simulink model "simulateur_pendule1"  (R2019b)
settings: Solver=VariableStepAuto  StartTime=0.0  StopTime=30.0  RelTol=1e-3
settings Model: Creator=Morin  LastModifiedBy=Morin

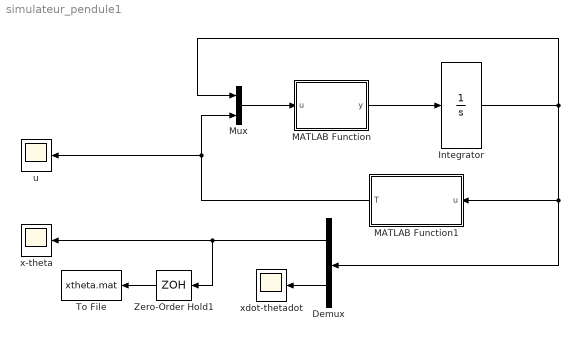
== system simulateur_pendule1 ==
  Demux : Demux  Outputs=2
  Integrator : Integrator  InitialCondition=[0;0.3;0;0]
  MATLAB Function : MATLAB Function  TreatAsAtomicUnit=on
  MATLAB Function1 : MATLAB Function  TreatAsAtomicUnit=on
  Mux : Mux  Inputs=2
  To File : ToFile  Filename=xtheta.mat  SaveFormat=Timeseries  SampleTime=0.01
  Zero-Order Hold1 : ZeroOrderHold  SampleTime=0.01
  u : Scope
  x-theta : Scope
  xdot-thetadot : Scope
  wires:
  MATLAB Function/1(y) -> Integrator/1
  Integrator/1 -> Mux/1, Demux/1, MATLAB Function1/1(u)
  Mux/1 -> MATLAB Function/1(u)
  Demux/1 -> Zero-Order Hold1/1, x-theta/1
  Demux/2 -> xdot-thetadot/1
  MATLAB Function1/1(T) -> u/1, Mux/2
  Zero-Order Hold1/1 -> To File/1

== matlab function simulateur_pendule1/MATLAB Function1 ==
  data: u input; T output
function T = commande(u)
% Fonction qui calcule la commande T

% Définition des états
x= u(1);
theta= u(2);
xdot= u(3);
thetadot=u(4);

% Definition des paramètres du système
m=0.2; % masse de la barre
M=1; % masse totale (chariot + barre)
l= 0.2 % demi-longueur de la barre
J=  m*l^2/3; % inertie de la barre
g= 9.81; % cste de gravité
mu= 0.005; % coeff. de frottement visqueux barre
tau= 0.2; % coeff. de frottement visqueux chariot

% Calcul de la commande
question= 1;
if question==1 % Stabilisation theta
    T_c= 0;
    T= tau*xdot+ T_c;
else % Stabilisation x et theta, méthode LQR
    T= 0;

end;

== matlab function simulateur_pendule1/MATLAB Function ==
  data: u input; y output
function y = dynamique(u)
% fonction définissant la dynamique du système: renvoie f(X,U) avec X
% l'état, et U la variable de commande physique (composante T de la force
% appliquée au chariot)

x= u(1); %position du chariot
theta= u(2); %inclinaison de la barre
xdot= u(3); % vitesse du chariot
thetadot= u(4); % vitesse angulaire de la barre
T= u(5); % force appliquée au chariot

% Defintion des paramètres du système
m= 0.2; % masse de la barre
M= 1; % masse totale (chariot + barre)
l= 0.2 % demi-longueur de la barre
J=  m*l^2/3; % inertie de la barre
g= 9.81; % cste de gravité
mu= 0.005; % coeff. de frottement visqueux barre
tau= 0.2; % coeff. de frottement visqueux chariot

% Calcul des dérivées secondes
Delta_theta= M*(J+m*l^2)-m^2*l^2*(cos(theta))^2;
xthetaddot=1/Delta_theta*[J+m*l^2 -m*l*cos(theta);-m*l*cos(theta) M]*...
    [T+m*l*thetadot^2*sin(theta)-tau*xdot;m*g*l*sin(theta)-mu*thetadot];
%Calcul de f
y = [xdot;thetadot;xthetaddot];
